simulink model "PUIOModel"  (R2017a)
settings: Solver=VariableStepAuto  StartTime=0.0  StopTime=tEnd  RelTol=1e-3  EnableMultiTasking=on
values from neighbouring files (symbols this model uses):
  A = [-1 1 1;1 -2 0;0 1 -3]    [ExampleActuator.m]    (also in ExamplePIUIO.m = [-2 0 1;0 -1 1;1 2 -3]; NewExampleActuator.m; Simulation.m; SinousidPIUIO.m)
  B = [1;1;0]    [ExampleActuator.m]    (also in ExamplePIUIO.m = [1;0;1]; NewExampleActuator.m; Simulation.m; SinousidPIUIO.m)
  C = [1 0 0;0 1 0]    [ExampleActuator.m]    (also in ExamplePIUIO.m = [1 2 3;0 1 2]; NewExampleActuator.m = [1 0 1;0 1 0]; Simulation.m = [1 0 1;0 1 0]; SinousidPIUIO.m = [1 0 1;0 1 0])
  d = dTS.Values.Data    [ExampleActuator.m]    (also in ExamplePIUIO.m; NewExampleActuator.m = 2; Simulation.m; SinousidPIUIO.m = 1)
  Ed = [1;0;0]    [ExampleActuator.m]    (also in ExamplePIUIO.m = [1;1;0]; NewExampleActuator.m; Simulation.m; SinousidPIUIO.m = [1;0;1])
  F = A1 - G1*C    [ExampleActuator.m]    (also in ExamplePIUIO.m = A1-G1*C; NewExampleActuator.m; PUIOfinder.m; SinousidPIUIO.m = A1-G1*C)
  G = G1 + A1*N - G1*C*N    [ExampleActuator.m]    (also in ExamplePIUIO.m = G1+G2; NewExampleActuator.m; PUIOfinder.m; SinousidPIUIO.m = G1+G2)
  H = T*B    [ExampleActuator.m]    (also in ExamplePIUIO.m; NewExampleActuator.m; PUIOfinder.m; SinousidPIUIO.m)
  M = eye(size(A))    [ExampleActuator.m]    (also in NewExampleActuator.m; PUIOfinder.m)
  N = Ed* pinv(C*Ed)    [ExampleActuator.m]    (also in ExamplePIUIO.m; NewExampleActuator.m; PUIOfinder.m = E* pinv(C*E); SinousidPIUIO.m)
  Ndhat = pinv(C*Ed)    [ExampleActuator.m]    (also in NewExampleActuator.m; Simulation.m = pinv(Caug*Eaug))
  x0 = [1;2;3]    [ExampleActuator.m]    (also in ExamplePIUIO.m; NewExampleActuator.m; Simulation.m; SinousidPIUIO.m)
  z0 = [0.1;0.2;0.3]    [ExampleActuator.m]    (also in ExamplePIUIO.m = xhat0; NewExampleActuator.m = [0.1,.2,0.3]; Simulation.m = [0.1;0.2;0.3;0.4;0.5]; SinousidPIUIO.m = xhat0)
settings Model: Creator=amirreza513  LastModifiedBy=amirreza513
settings OptimizationCC: LifeSpan=inf
settings DebuggingCC: SFUnexpectedBacktrackingDiag=warning  SFNoUnconditionalDefaultTransitionDiag=warning  SFExecutionAtInitializationDiag=none
settings GRTTargetCC: TargetLangStandard=C89/C90 (ANSI)  GeneratePreprocessorConditionals=Disable all
settings ConfigComp: CovMetricSettings=dw  CovHtmlReporting=on  CovSaveCumulativeToWorkspaceVar=on  CovSaveSingleToWorkspaceVar=on  CovExternalEMLEnable=off

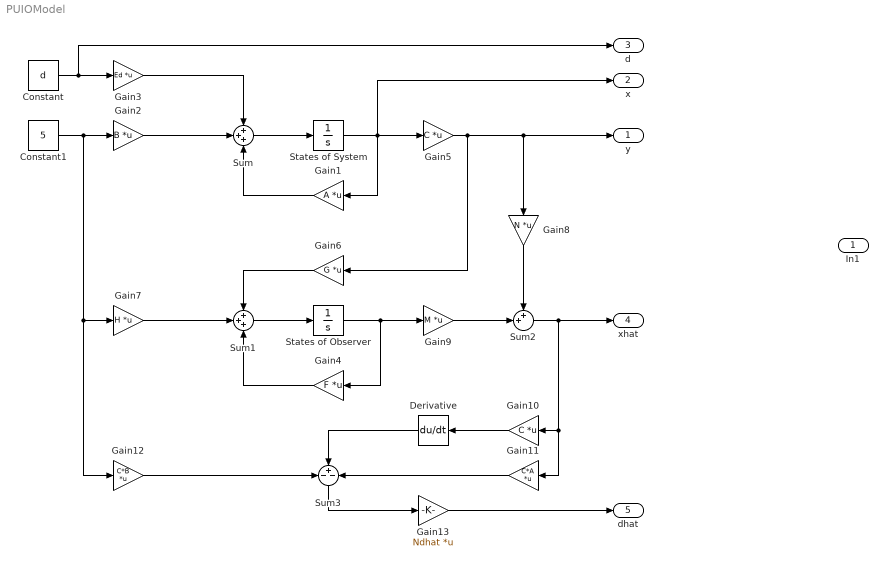
== system PUIOModel ==
  In1 : Inport
  Constant : Constant  Value=d
  Constant1 : Constant  Value=5
  Derivative : Derivative  CoefficientInTFapproximation=0
  Gain1 : Gain  Gain=A  Multiplication=Matrix(K*u) (u vector)
  Gain10 : Gain  Gain=C  Multiplication=Matrix(K*u) (u vector)
  Gain11 : Gain  Gain=C*A  Multiplication=Matrix(K*u) (u vector)
  Gain12 : Gain  Gain=C*B  Multiplication=Matrix(K*u) (u vector)
  Gain13 : Gain  Gain=Ndhat  Multiplication=Matrix(K*u) (u vector)
  Gain2 : Gain  Gain=B  Multiplication=Matrix(K*u) (u vector)
  Gain3 : Gain  Gain=Ed  Multiplication=Matrix(K*u) (u vector)
  Gain4 : Gain  Gain=F  Multiplication=Matrix(K*u) (u vector)
  Gain5 : Gain  Gain=C  Multiplication=Matrix(K*u) (u vector)
  Gain6 : Gain  Gain=G  Multiplication=Matrix(K*u) (u vector)
  Gain7 : Gain  Gain=H  Multiplication=Matrix(K*u) (u vector)
  Gain8 : Gain  Gain=N  Multiplication=Matrix(K*u) (u vector)
  Gain9 : Gain  Gain=M  Multiplication=Matrix(K*u) (u vector)
  States of Observer : Integrator  InitialCondition=z0
  States of System : Integrator  InitialCondition=x0
  Sum : Sum  Inputs=+++
  Sum1 : Sum  Inputs=+++
  Sum2 : Sum  Inputs=++|
  Sum3 : Sum  Inputs=-+-
  y : Outport
  x : Outport  Port=2
  d : Outport  Port=3
  xhat : Outport  Port=4
  dhat : Outport  Port=5
  wires:
  States of System/1 -> x/1, Gain5/1, Gain1/1
  Constant1/1 -> Gain12/1, Gain7/1, Gain2/1
  Gain2/1 -> Sum/2
  Constant/1 -> d/1, Gain3/1
  Sum/1 -> States of System/1
  Gain5/1 -> Gain6/1, Gain8/1, y/1
  Gain3/1 -> Sum/1
  Gain1/1 -> Sum/3
  Sum1/1 -> States of Observer/1
  States of Observer/1 -> Gain9/1, Gain4/1
  Gain6/1 -> Sum1/1
  Gain7/1 -> Sum1/2
  Gain4/1 -> Sum1/3
  Gain8/1 -> Sum2/1
  Gain9/1 -> Sum2/2
  Gain10/1 -> Derivative/1
  Sum2/1 -> Gain11/1, Gain10/1, xhat/1
  Gain12/1 -> Sum3/1
  Derivative/1 -> Sum3/2
  Gain11/1 -> Sum3/3
  Sum3/1 -> Gain13/1
  Gain13/1 -> dhat/1
